simulink model "chap7_4sim"  (Simulink 7.7)
settings: Solver=ode45  StartTime=0.0  StopTime=10  FixedStep=0.00000010  RelTol=1e-3
settings Model: Creator=ljk  LastModifiedBy=ljk  ExtModeTrigMode=oneshot  ExtModeArmWhenConnect=off
settings DataIOCC: LimitDataPoints=off  SignalLoggingName=sigsOut
settings OptimizationCC: BooleanDataType=off
settings DebuggingCC: SaveWithParameterizedLinksMsg=none  SignalResolutionControl=TryResolveAllWithWarning  SolverPrmCheckMsg=none  MultiTaskDSMMsg=warning  MultiTaskCondExecSysMsg=none  StrictBusMsg=None
settings HardwareCC: TargetUnknown=on
settings RTWCC: IncludeERTFirstTime=on
settings CodeAppCC: CustomSymbolStrType=$N$R$M_T

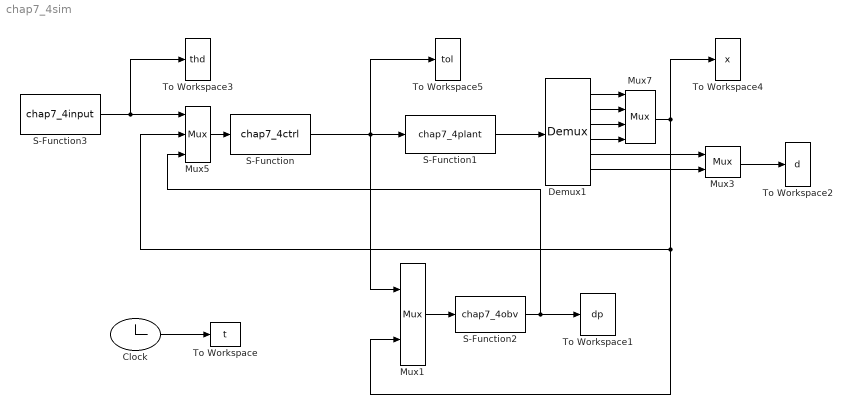
== system chap7_4sim ==
  Clock : Clock
  Demux1 : Demux  Outputs=6
  Mux1 : Mux  Inputs=2
  Mux3 : Mux  Inputs=2
  Mux5 : Mux  Inputs=3
  Mux7 : Mux
  S-Function : S-Function  FunctionName=chap7_4ctrl  EnableBusSupport=off
  S-Function1 : S-Function  FunctionName=chap7_4plant  EnableBusSupport=off
  S-Function2 : S-Function  FunctionName=chap7_4obv  EnableBusSupport=off
  S-Function3 : S-Function  FunctionName=chap7_4input  EnableBusSupport=off
  To Workspace : ToWorkspace  VariableName=t  SampleTime=-1  SaveFormat=Array
  To Workspace1 : ToWorkspace  VariableName=dp  SampleTime=-1  SaveFormat=Array
  To Workspace2 : ToWorkspace  VariableName=d  SampleTime=-1  SaveFormat=Array
  To Workspace3 : ToWorkspace  VariableName=thd  SampleTime=-1  SaveFormat=Array
  To Workspace4 : ToWorkspace  VariableName=x  SampleTime=-1  SaveFormat=Array
  To Workspace5 : ToWorkspace  VariableName=tol  SampleTime=-1  SaveFormat=Array
  wires:
  Clock/1 -> To Workspace/1
  Mux1/1 -> S-Function2/1
  S-Function3/1 -> Mux5/1, To Workspace3/1
  S-Function1/1 -> Demux1/1
  Demux1/1 -> Mux7/1
  Demux1/2 -> Mux7/2
  Demux1/3 -> Mux7/3
  Demux1/4 -> Mux7/4
  Mux7/1 -> To Workspace4/1, Mux5/2, Mux1/2
  Demux1/5 -> Mux3/1
  Demux1/6 -> Mux3/2
  Mux3/1 -> To Workspace2/1
  Mux5/1 -> S-Function/1
  S-Function/1 -> To Workspace5/1, S-Function1/1, Mux1/1
  S-Function2/1 -> Mux5/3, To Workspace1/1
